simulink model "obwod_naprowadzania_JW"  (Simulink 10.2)
settings: Solver=VariableStepAuto  StartTime=0.0  StopTime=t_sim  MaxStep=0.005  EnableMultiTasking=on
values from neighbouring files (symbols this model uses):
  B_cel0 = deg2rad(-180)    [progaram_symulacyjny.m]
  E_cel0 = deg2rad(0)    [progaram_symulacyjny.m]
  v0 = 300    [progaram_symulacyjny.m]
  x0 = sqrt(23500^2-y0^2-z0^2)+v0*40    [progaram_symulacyjny.m]
  y0 = 0    [progaram_symulacyjny.m]
  z0 = 7000    [progaram_symulacyjny.m]
undefined symbols (not defined in the file or in its folder): beta_0_prim_srcp, caL, epsilon_0_prim_srcp, Fm, Fs, g, h_uwk, Im0, Im1, Is0, Is1, R, RB, RBC, RC, RE, REC, S, tm, ts, tster
libraries: simulink_extras x6, simulink x3
(part 2 of 2)

== system obwod_naprowadzania_JW/MODEL RAKIETY/Zaleznosci na skladowe sil i momentow aerodynamicznych/cx0(t) ==
  in_1 : Inport
  Constant : Constant  Value=ts
  Constant1 : Constant  Value=0.195
  Constant2 : Constant  Value=3.2
  Constant3 : Constant  Value=ts+tm
  Constant4 : Constant  Value=0.15
  Logical Operator : Logic
  Product : Product  InputSameDT=on  RndMeth=Zero  SaturateOnIntegerOverflow=on  OutDataTypeStr=Inherit: Same as first input
  Product1 : Product  InputSameDT=on  RndMeth=Zero  SaturateOnIntegerOverflow=on  OutDataTypeStr=Inherit: Same as first input
  Product2 : Product  InputSameDT=on  RndMeth=Zero  SaturateOnIntegerOverflow=on  OutDataTypeStr=Inherit: Same as first input
  Relational Operator : RelationalOperator  Operator=<=  RndMeth=Nearest  InputSameDT=on
  Relational Operator1 : RelationalOperator  Operator=>  RndMeth=Nearest  InputSameDT=on
  Relational Operator2 : RelationalOperator  Operator=<=  RndMeth=Nearest  InputSameDT=on
  Relational Operator3 : RelationalOperator  Operator=>  RndMeth=Nearest  InputSameDT=on
  Sum : Sum  Inputs=+++  InputSameDT=on  SaturateOnIntegerOverflow=on  OutDataTypeStr=Inherit: Same as first input
  out_1 : Outport
  wires:
  Sum/1 -> out_1/1
  Logical Operator/1 -> Product1/1
  Constant3/1 -> Relational Operator2/2, Relational Operator3/2
  Relational Operator2/1 -> Logical Operator/2
  Relational Operator1/1 -> Logical Operator/1
  Constant/1 -> Relational Operator1/2, Relational Operator/2
  in_1/1 -> Relational Operator1/1, Relational Operator2/1, Relational Operator3/1, Relational Operator/1
  Relational Operator/1 -> Product/2
  Constant2/1 -> Product/1
  Product/1 -> Sum/1
  Constant4/1 -> Product1/2
  Product1/1 -> Sum/2
  Relational Operator3/1 -> Product2/1
  Constant1/1 -> Product2/2
  Product2/1 -> Sum/3

== system obwod_naprowadzania_JW/MODEL RAKIETY/Zaleznosci na skladowe sil i momentow aerodynamicznych/cxi(t) ==
  in_1 : Inport
  Constant : Constant  Value=ts
  Constant2 : Constant  Value=18.9
  Constant4 : Constant  Value=5.9
  Product : Product  InputSameDT=on  RndMeth=Zero  SaturateOnIntegerOverflow=on  OutDataTypeStr=Inherit: Same as first input
  Product1 : Product  InputSameDT=on  RndMeth=Zero  SaturateOnIntegerOverflow=on  OutDataTypeStr=Inherit: Same as first input
  Relational Operator : RelationalOperator  Operator=<=  RndMeth=Nearest  InputSameDT=on
  Relational Operator1 : RelationalOperator  Operator=>  RndMeth=Nearest  InputSameDT=on
  Sum : Sum  InputSameDT=on  SaturateOnIntegerOverflow=on  OutDataTypeStr=Inherit: Same as first input
  out_1 : Outport
  wires:
  Product1/1 -> Sum/2
  Constant2/1 -> Product/1
  Relational Operator/1 -> Product/2
  in_1/1 -> Relational Operator/1, Relational Operator1/1
  Constant/1 -> Relational Operator/2, Relational Operator1/2
  Relational Operator1/1 -> Product1/1
  Sum/1 -> out_1/1
  Constant4/1 -> Product1/2
  Product/1 -> Sum/1

== system obwod_naprowadzania_JW/MODEL RAKIETY/Zaleznosci na skladowe sil i momentow aerodynamicznych/cy ==
  in_1 : Inport
  Fcn : Fcn  Expr=-u(3)*u(2)+u(4)*u(8)
  out_1 : Outport
  wires:
  Fcn/1 -> out_1/1
  in_1/1 -> Fcn/1

== system obwod_naprowadzania_JW/MODEL RAKIETY/Zaleznosci na skladowe sil i momentow aerodynamicznych/cz ==
  in_1 : Inport
  Fcn : Fcn  Expr=u(3)*u(1)+u(4)*u(7)
  out_1 : Outport
  wires:
  in_1/1 -> Fcn/1
  Fcn/1 -> out_1/1

== system obwod_naprowadzania_JW/MODEL RAKIETY/Zaleznosci na skladowe sil i momentow aerodynamicznych/cz_alfa(Ma) ==
  in_1 : Inport
  Fcn : Fcn  Expr=(0.40625-0.051875*u(1))*(180/pi)
  out_1 : Outport
  wires:
  Fcn/1 -> out_1/1
  in_1/1 -> Fcn/1

== system obwod_naprowadzania_JW/MODEL RAKIETY/Zaleznosci na skladowe sil i momentow aerodynamicznych/cz_delta(Ma) ==
  in_1 : Inport
  Fcn : Fcn  Expr=(0.02362-0.004686*u(1))*(180/pi)
  out_1 : Outport
  wires:
  in_1/1 -> Fcn/1
  Fcn/1 -> out_1/1

== system obwod_naprowadzania_JW/MODEL RAKIETY/Zaleznosci na skladowe sil i momentow aerodynamicznych/xsm(t) ==
  in_1 : Inport
  Constant : Constant  Value=ts
  Constant1 : Constant  Value=2.385
  Constant3 : Constant  Value=ts+tm
  Fcn : Fcn  Expr=3.984-((3.984-3.586)/ts)*u(1)
  Fcn1 : Fcn  Expr=2.715-((2.715-2.385)/tm)*(u(1)-ts)
  Logical Operator : Logic
  Product : Product  InputSameDT=on  RndMeth=Zero  SaturateOnIntegerOverflow=on  OutDataTypeStr=Inherit: Same as first input
  Product1 : Product  InputSameDT=on  RndMeth=Zero  SaturateOnIntegerOverflow=on  OutDataTypeStr=Inherit: Same as first input
  Product2 : Product  InputSameDT=on  RndMeth=Zero  SaturateOnIntegerOverflow=on  OutDataTypeStr=Inherit: Same as first input
  Relational Operator : RelationalOperator  Operator=<=  RndMeth=Nearest  InputSameDT=on
  Relational Operator1 : RelationalOperator  Operator=>  RndMeth=Nearest  InputSameDT=on
  Relational Operator2 : RelationalOperator  Operator=<=  RndMeth=Nearest  InputSameDT=on
  Relational Operator3 : RelationalOperator  Operator=>  RndMeth=Nearest  InputSameDT=on
  Sum : Sum  Inputs=+++  InputSameDT=on  SaturateOnIntegerOverflow=on  OutDataTypeStr=Inherit: Same as first input
  out_1 : Outport
  wires:
  Product2/1 -> Sum/3
  Constant1/1 -> Product2/2
  Relational Operator3/1 -> Product2/1
  Product1/1 -> Sum/2
  Fcn1/1 -> Product1/2
  Product/1 -> Sum/1
  Fcn/1 -> Product/1
  Relational Operator/1 -> Product/2
  in_1/1 -> Fcn/1, Relational Operator/1, Relational Operator3/1, Fcn1/1, Relational Operator2/1, Relational Operator1/1
  Constant/1 -> Relational Operator/2, Relational Operator1/2
  Relational Operator1/1 -> Logical Operator/1
  Relational Operator2/1 -> Logical Operator/2
  Constant3/1 -> Relational Operator3/2, Relational Operator2/2
  Logical Operator/1 -> Product1/1
  Sum/1 -> out_1/1

== system obwod_naprowadzania_JW/MODEL RAKIETY/Zaleznosci na skladowe sil i momentow aerodynamicznych/xsp(t) ==
  in_1 : Inport
  Constant : Constant  Value=ts
  Constant2 : Constant  Value=3.95
  Constant4 : Constant  Value=3
  Product : Product  InputSameDT=on  RndMeth=Zero  SaturateOnIntegerOverflow=on  OutDataTypeStr=Inherit: Same as first input
  Product1 : Product  InputSameDT=on  RndMeth=Zero  SaturateOnIntegerOverflow=on  OutDataTypeStr=Inherit: Same as first input
  Relational Operator : RelationalOperator  Operator=<=  RndMeth=Nearest  InputSameDT=on
  Relational Operator1 : RelationalOperator  Operator=>  RndMeth=Nearest  InputSameDT=on
  Sum : Sum  InputSameDT=on  SaturateOnIntegerOverflow=on  OutDataTypeStr=Inherit: Same as first input
  out_1 : Outport
  wires:
  Product/1 -> Sum/1
  Constant4/1 -> Product1/2
  Sum/1 -> out_1/1
  Relational Operator1/1 -> Product1/1
  Constant/1 -> Relational Operator1/2, Relational Operator/2
  in_1/1 -> Relational Operator1/1, Relational Operator/1
  Relational Operator/1 -> Product/2
  Constant2/1 -> Product/1
  Product1/1 -> Sum/2

== system obwod_naprowadzania_JW/MODEL UWK/Komendy Kierowania Waskie Pasmo/Subsystem ==
  note: f_hr1w
  hl1 : Inport
  Constant : Constant  Value=11.857142857
  Constant1 : Constant  Value=0.14
  Memory : Memory
  Product : Product  InputSameDT=on  RndMeth=Zero  SaturateOnIntegerOverflow=on  OutDataTypeStr=Inherit: Same as first input
  Product1 : Product  Inputs=*/  InputSameDT=on  RndMeth=Zero  SaturateOnIntegerOverflow=on  OutDataTypeStr=Inherit: Same as first input
  Product2 : Product  InputSameDT=on  RndMeth=Zero  SaturateOnIntegerOverflow=on  OutDataTypeStr=Inherit: Same as first input
  Product3 : Product  InputSameDT=on  RndMeth=Zero  SaturateOnIntegerOverflow=on  OutDataTypeStr=Inherit: Same as first input
  Sum : Sum  Inputs=+-  InputSameDT=on  SaturateOnIntegerOverflow=on  OutDataTypeStr=Inherit: Same as first input
  Sum1 : Sum  InputSameDT=on  SaturateOnIntegerOverflow=on  OutDataTypeStr=Inherit: Same as first input
  Sum2 : Sum  Inputs=+-  InputSameDT=on  SaturateOnIntegerOverflow=on  OutDataTypeStr=Inherit: Same as first input
  h_uwk : Constant  Value=h_uwk
  liczUR : Constant
  h1rw : Outport
  wires:
  Constant/1 -> Product/2
  Product/1 -> Sum/1, Sum2/1
  Sum/1 -> Product1/1
  Constant1/1 -> Product1/2
  Sum1/1 -> Sum/2, Memory/1, Sum2/2
  h_uwk/1 -> Product2/2
  Product1/1 -> Product2/1
  Product2/1 -> Sum1/2
  Sum2/1 -> Product3/1
  liczUR/1 -> Product3/2
  Product3/1 -> h1rw/1
  hl1/1 -> Product/1
  Memory/1 -> Sum1/1

== system obwod_naprowadzania_JW/MODEL UWK/Komendy Kierowania Waskie Pasmo/Subsystem1 ==
  hl2 : Inport
  Constant : Constant  Value=11.857142857
  Constant1 : Constant  Value=0.14
  Memory : Memory
  Product : Product  InputSameDT=on  RndMeth=Zero  SaturateOnIntegerOverflow=on  OutDataTypeStr=Inherit: Same as first input
  Product1 : Product  Inputs=*/  InputSameDT=on  RndMeth=Zero  SaturateOnIntegerOverflow=on  OutDataTypeStr=Inherit: Same as first input
  Product2 : Product  InputSameDT=on  RndMeth=Zero  SaturateOnIntegerOverflow=on  OutDataTypeStr=Inherit: Same as first input
  Product3 : Product  InputSameDT=on  RndMeth=Zero  SaturateOnIntegerOverflow=on  OutDataTypeStr=Inherit: Same as first input
  Sum : Sum  Inputs=+-  InputSameDT=on  SaturateOnIntegerOverflow=on  OutDataTypeStr=Inherit: Same as first input
  Sum1 : Sum  InputSameDT=on  SaturateOnIntegerOverflow=on  OutDataTypeStr=Inherit: Same as first input
  Sum2 : Sum  Inputs=+-  InputSameDT=on  SaturateOnIntegerOverflow=on  OutDataTypeStr=Inherit: Same as first input
  h_uwk : Constant  Value=h_uwk
  liczUR : Constant
  h2rw : Outport
  wires:
  hl2/1 -> Product/1
  Product3/1 -> h2rw/1
  liczUR/1 -> Product3/2
  Sum2/1 -> Product3/1
  Product2/1 -> Sum1/2
  Product1/1 -> Product2/1
  h_uwk/1 -> Product2/2
  Sum1/1 -> Sum2/2, Sum/2, Memory/1
  Constant1/1 -> Product1/2
  Sum/1 -> Product1/1
  Product/1 -> Sum2/1, Sum/1
  Constant/1 -> Product/2
  Memory/1 -> Sum1/1

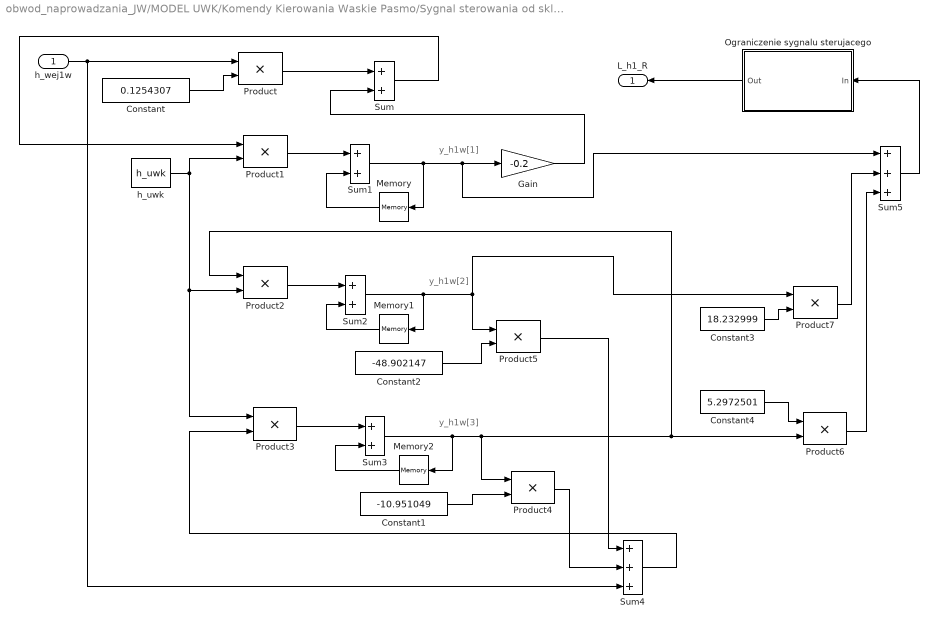
== system obwod_naprowadzania_JW/MODEL UWK/Komendy Kierowania Waskie Pasmo/Sygnal sterowania od skladowej liniowej ==
  note: y_h1w[1]
  note: y_h1w[2]
  note: y_h1w[3]
  h_wej1w : Inport
  Constant : Constant  Value=0.1254307
  Constant1 : Constant  Value=-10.951049
  Constant2 : Constant  Value=-48.902147
  Constant3 : Constant  Value=18.232999
  Constant4 : Constant  Value=5.2972501
  Gain : Gain  Gain=-0.2  SaturateOnIntegerOverflow=on  OutDataTypeStr=Inherit: Same as input  ParamDataTypeStr=Inherit: Same as input
  Memory : Memory
  Memory1 : Memory
  Memory2 : Memory
  Ograniczenie sygnalu sterujacego : Subsystem
  Product{,1..7} (8 alike) : Product  InputSameDT=on  RndMeth=Zero  SaturateOnIntegerOverflow=on  OutDataTypeStr=Inherit: Same as first input
  Sum{,1..3} (4 alike) : Sum  InputSameDT=on  SaturateOnIntegerOverflow=on  OutDataTypeStr=Inherit: Same as first input
  Sum4 : Sum  Inputs=+++  InputSameDT=on  SaturateOnIntegerOverflow=on  OutDataTypeStr=Inherit: Same as first input
  Sum5 : Sum  Inputs=+++  InputSameDT=on  SaturateOnIntegerOverflow=on  OutDataTypeStr=Inherit: Same as first input
  h_uwk : Constant  Value=h_uwk
  L_h1_R : Outport
  wires:
  h_wej1w/1 -> Product/1, Sum4/3
  Constant/1 -> Product/2
  Sum/1 -> Product1/1
  Product/1 -> Sum/1
  Sum1/1 -> Gain/1, Sum5/1, Memory/1
  h_uwk/1 -> Product1/2, Product2/2, Product3/1
  Product1/1 -> Sum1/1
  Gain/1 -> Sum/2
  Sum2/1 -> Product5/1, Product7/1, Memory1/1
  Product2/1 -> Sum2/1
  Sum3/1 -> Product4/1, Product2/1, Product6/2, Memory2/1
  Product3/1 -> Sum3/1
  Constant1/1 -> Product4/2
  Constant2/1 -> Product5/2
  Product5/1 -> Sum4/1
  Product4/1 -> Sum4/2
  Sum4/1 -> Product3/2
  Constant3/1 -> Product7/2
  Product7/1 -> Sum5/2
  Sum5/1 -> Ograniczenie sygnalu sterujacego/1(In)
  Constant4/1 -> Product6/1
  Product6/1 -> Sum5/3
  Ograniczenie sygnalu sterujacego/1(Out) -> L_h1_R/1
  Memory/1 -> Sum1/2
  Memory1/1 -> Sum2/2
  Memory2/1 -> Sum3/2

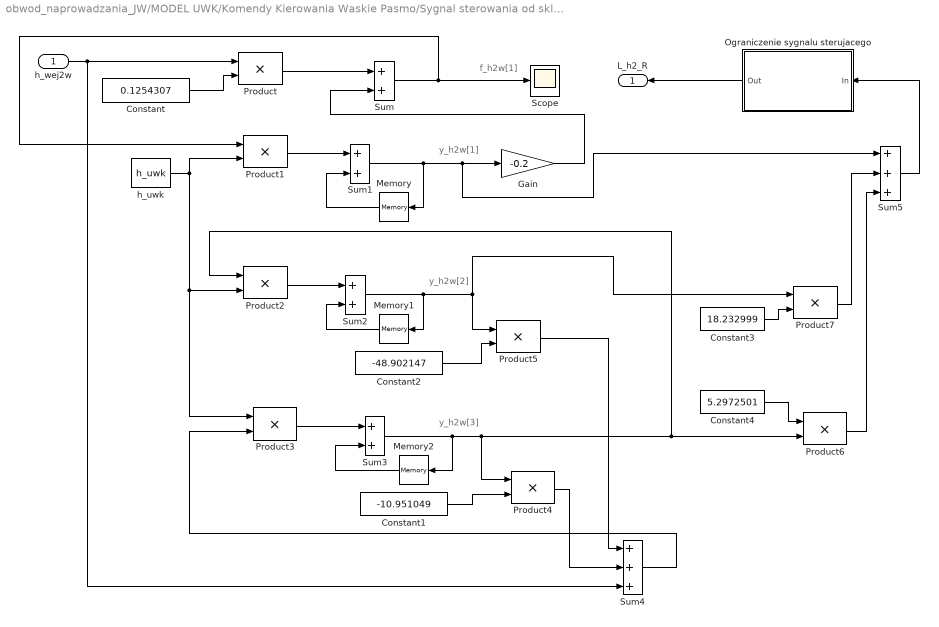
== system obwod_naprowadzania_JW/MODEL UWK/Komendy Kierowania Waskie Pasmo/Sygnal sterowania od skladowej liniowej1 ==
  note: f_h2w[1]
  note: y_h2w[3]
  note: y_h2w[2]
  note: y_h2w[1]
  h_wej2w : Inport
  Constant : Constant  Value=0.1254307
  Constant1 : Constant  Value=-10.951049
  Constant2 : Constant  Value=-48.902147
  Constant3 : Constant  Value=18.232999
  Constant4 : Constant  Value=5.2972501
  Gain : Gain  Gain=-0.2  SaturateOnIntegerOverflow=on  OutDataTypeStr=Inherit: Same as input  ParamDataTypeStr=Inherit: Same as input
  Memory : Memory
  Memory1 : Memory
  Memory2 : Memory
  Ograniczenie sygnalu sterujacego : Subsystem
  Product{,1..7} (8 alike) : Product  InputSameDT=on  RndMeth=Zero  SaturateOnIntegerOverflow=on  OutDataTypeStr=Inherit: Same as first input
  Scope : Scope
  Sum{,1..3} (4 alike) : Sum  InputSameDT=on  SaturateOnIntegerOverflow=on  OutDataTypeStr=Inherit: Same as first input
  Sum4 : Sum  Inputs=+++  InputSameDT=on  SaturateOnIntegerOverflow=on  OutDataTypeStr=Inherit: Same as first input
  Sum5 : Sum  Inputs=+++  InputSameDT=on  SaturateOnIntegerOverflow=on  OutDataTypeStr=Inherit: Same as first input
  h_uwk : Constant  Value=h_uwk
  L_h2_R : Outport
  wires:
  Memory2/1 -> Sum3/2
  Memory1/1 -> Sum2/2
  Memory/1 -> Sum1/2
  Ograniczenie sygnalu sterujacego/1(Out) -> L_h2_R/1
  Product6/1 -> Sum5/3
  Constant4/1 -> Product6/1
  Sum5/1 -> Ograniczenie sygnalu sterujacego/1(In)
  Product7/1 -> Sum5/2
  Constant3/1 -> Product7/2
  Sum4/1 -> Product3/2
  Product4/1 -> Sum4/2
  Product5/1 -> Sum4/1
  Constant2/1 -> Product5/2
  Constant1/1 -> Product4/2
  Product3/1 -> Sum3/1
  Sum3/1 -> Memory2/1, Product4/1, Product6/2, Product2/1
  Product2/1 -> Sum2/1
  Sum2/1 -> Memory1/1, Product7/1, Product5/1
  Gain/1 -> Sum/2
  Product1/1 -> Sum1/1
  h_uwk/1 -> Product3/1, Product2/2, Product1/2
  Sum1/1 -> Memory/1, Sum5/1, Gain/1
  Product/1 -> Sum/1
  Sum/1 -> Scope/1, Product1/1
  Constant/1 -> Product/2
  h_wej2w/1 -> Sum4/3, Product/1

== system obwod_naprowadzania_JW/MODEL UWK/Odchyki/gamma_R ==
  azymut : Inport
  elewacja : Inport  Port=2
  Derivative : Derivative
  Memory : Memory
  Product : Product  Inputs=4  InputSameDT=on  RndMeth=Zero  SaturateOnIntegerOverflow=on  OutDataTypeStr=Inherit: Same as first input
  Sum4 : Sum  Inputs=+-  InputSameDT=on  SaturateOnIntegerOverflow=on  OutDataTypeStr=Inherit: Same as first input
  Trigonometric Function : Trigonometry
  h_uwk : Constant  Value=h_uwk
  tster : Step  Time=tster  SampleTime=0
  gammaR : Outport
  wires:
  elewacja/1 -> Trigonometric Function/1
  Trigonometric Function/1 -> Product/2
  azymut/1 -> Derivative/1
  Derivative/1 -> Product/1
  h_uwk/1 -> Product/3
  Product/1 -> Sum4/2
  Memory/1 -> Sum4/1
  tster/1 -> Product/4
  Sum4/1 -> Memory/1, gammaR/1

== system obwod_naprowadzania_JW/MODEL CELU/Model samolotu/Ogranicznik przeciążenia  wypadkowego (max 9g)/sprzężenie zwrotne (wzrost prędkości o zadaną wartość) ==
  Fcn(n) : Inport
  u : Inport  Port=2
  -Fcn(n) : Inport  Port=3
  y : Inport  Port=4
  Add : Sum  Inputs=+-
  Add1 : Sum
  Gain1 : Gain  Gain=-1
  Integrator : Integrator
  Integrator1 : Integrator
  Switch : Switch  Criteria=u2 > Threshold  Threshold=0.000001
  Switch1 : Switch  Criteria=u2 > Threshold  Threshold=0.000001
  Zero : Constant  Value=0  OutDataTypeStr=Inherit: Inherit via back propagation
  Zero1 : Constant  Value=0  OutDataTypeStr=Inherit: Inherit via back propagation
  sprz : Outport
  wires:
  Integrator/1 -> Add/2
  Add/1 -> Gain1/1, Switch/2
  Zero/1 -> Switch/3
  Integrator1/1 -> Add/1
  Gain1/1 -> Switch1/2
  Zero1/1 -> Switch1/3
  Switch/1 -> Add1/1
  Switch1/1 -> Add1/2
  Fcn(n)/1 -> Switch/1
  u/1 -> Integrator1/1
  y/1 -> Integrator/1
  Add1/1 -> sprz/1
  -Fcn(n)/1 -> Switch1/1

== system obwod_naprowadzania_JW/MODEL CELU/Model samolotu/Ogranicznik przeciążenia azymut (max 4g)/sprzężenie zwrotne (skręt o zadany kąt) ==
  u : Inport
  Fcn(v) : Inport  Port=2
  y : Inport  Port=3
  Add : Sum  Inputs=+-
  Add1 : Sum
  Gain1 : Gain  Gain=-1
  Gain2 : Gain  Gain=-1
  Integrator : Integrator
  Integrator1 : Integrator
  Switch : Switch  Criteria=u2 > Threshold  Threshold=0.000001
  Switch1 : Switch  Criteria=u2 > Threshold  Threshold=0.000001
  Zero : Constant  Value=0  OutDataTypeStr=Inherit: Inherit via back propagation
  Zero1 : Constant  Value=0  OutDataTypeStr=Inherit: Inherit via back propagation
  sprz : Outport
  wires:
  Integrator/1 -> Add/2
  Add/1 -> Gain1/1, Switch/2
  Zero/1 -> Switch/3
  Integrator1/1 -> Add/1
  Gain1/1 -> Switch1/2
  Zero1/1 -> Switch1/3
  Switch/1 -> Add1/1
  Gain2/1 -> Switch1/1
  Switch1/1 -> Add1/2
  Fcn(v)/1 -> Switch/1, Gain2/1
  u/1 -> Integrator1/1
  y/1 -> Integrator/1
  Add1/1 -> sprz/1

== system obwod_naprowadzania_JW/MODEL CELU/Model samolotu/Ogranicznik przeciążenia elewacja (max 8g)/sprzężenie zwrotne (skręt o zadany kąt) ==
  u : Inport
  Fcn(v) : Inport  Port=2
  y : Inport  Port=3
  Add : Sum  Inputs=+-
  Add1 : Sum
  Gain1 : Gain  Gain=-1
  Gain2 : Gain  Gain=-1
  Integrator : Integrator
  Integrator1 : Integrator
  Switch : Switch  Criteria=u2 > Threshold  Threshold=0.000001
  Switch1 : Switch  Criteria=u2 > Threshold  Threshold=0.000001
  Zero : Constant  Value=0  OutDataTypeStr=Inherit: Inherit via back propagation
  Zero1 : Constant  Value=0  OutDataTypeStr=Inherit: Inherit via back propagation
  Out1 : Outport
  wires:
  Integrator/1 -> Add/2
  Add/1 -> Gain1/1, Switch/2
  Zero/1 -> Switch/3
  Integrator1/1 -> Add/1
  Gain1/1 -> Switch1/2
  Zero1/1 -> Switch1/3
  Switch/1 -> Add1/1
  Gain2/1 -> Switch1/1
  Switch1/1 -> Add1/2
  Fcn(v)/1 -> Switch/1, Gain2/1
  u/1 -> Integrator1/1
  y/1 -> Integrator/1
  Add1/1 -> Out1/1

== system obwod_naprowadzania_JW/MODEL RAKIETY/Zaleznosci na skladowe sil i momentow aerodynamicznych/PN-78/N-03100  /cisnienie ==
  H : Inport
  11000 > H >= 0 : Subsystem
  20000 > H >= 11000 : Subsystem
  32000 > H >= 20000 : Subsystem
  47000 > H >= 32000 : Subsystem
  51000 > H >= 47000 : Subsystem
  71000 > H >= 51000 : Subsystem
  80000 > H >= 71000 : Subsystem
  Sum : Sum  Inputs=+++++++  InputSameDT=on  SaturateOnIntegerOverflow=on  OutDataTypeStr=Inherit: Same as first input
  "cisnienie - p [Pa] " : Scope
  p : Outport
  wires:
  80000 > H >= 71000/1(Out1) -> Sum/7
  71000 > H >= 51000/1(Out1) -> Sum/6
  51000 > H >= 47000/1(Out1) -> Sum/5
  47000 > H >= 32000/1(Out1) -> Sum/4
  32000 > H >= 20000/1(Out1) -> Sum/3
  20000 > H >= 11000/1(Out1) -> Sum/2
  Sum/1 -> "cisnienie - p [Pa] "/1, p/1
  11000 > H >= 0/1(Out1) -> Sum/1
  H/1 -> 80000 > H >= 71000/1(In1), 71000 > H >= 51000/1(In1), 51000 > H >= 47000/1(In1), 47000 > H >= 32000/1(In1), 32000 > H >= 20000/1(In1), 20000 > H >= 11000/1(In1), 11000 > H >= 0/1(In1)

== system obwod_naprowadzania_JW/MODEL RAKIETY/Zaleznosci na skladowe sil i momentow aerodynamicznych/PN-78/N-03100  /gestosc ==
  note: wlasciwa stala gazowa - R
  p : Inport
  T : Inport  Port=2
  Math Function : Math  Operator=reciprocal  SignedPower=on  SaturateOnIntegerOverflow=on
  Product1 : Product  InputSameDT=on  RndMeth=Zero  SaturateOnIntegerOverflow=on  OutDataTypeStr=Inherit: Same as first input
  Product2 : Product  InputSameDT=on  RndMeth=Zero  SaturateOnIntegerOverflow=on  OutDataTypeStr=Inherit: Same as first input
  R [J/K*kg] [m2/K*s2] : Constant  Value=287.05287
  "gestosc [kg/m3] " : Scope
  gestosc : Outport
  wires:
  Product2/1 -> "gestosc [kg/m3] "/1, gestosc/1
  p/1 -> Product2/1
  Math Function/1 -> Product2/2
  Product1/1 -> Math Function/1
  T/1 -> Product1/1
  R [J/K*kg] [m2/K*s2]/1 -> Product1/2

== system obwod_naprowadzania_JW/MODEL RAKIETY/Zaleznosci na skladowe sil i momentow aerodynamicznych/PN-78/N-03100  /predkosc dzwieku ==
  note: wlasciwa stala gazowa - R
  note: wykladnik adiabaty - stosunek ciepla wlasciwego
      | powietrza przy stalym cisnieniu do jego ciepla
      | wlasciwego przy stalej objetosci
  note: temperatura termodynamiczna - T [K]
  T : Inport
  Math Function : Math  Operator=sqrt  SignedPower=on  SaturateOnIntegerOverflow=on
  Math Function1 : Math  Operator=sqrt  SignedPower=on  SaturateOnIntegerOverflow=on
  Product : Product  InputSameDT=on  RndMeth=Zero  SaturateOnIntegerOverflow=on  OutDataTypeStr=Inherit: Same as first input
  Product1 : Product  Inputs=3  InputSameDT=on  RndMeth=Zero  SaturateOnIntegerOverflow=on  OutDataTypeStr=Inherit: Same as first input
  R [J/K*kg] [m2/K*s2] : Constant  Value=287.05287
  k=Cp/Cv : Constant  Value=1.4
  "predkosc dzwieku - a [m/s] " : Scope
  predkosc dzwieku a [m/s] : Scope
  stala : Constant  Value=20.046796
  predkosc dzwieku : Outport
  wires:
  Product1/1 -> Math Function1/1
  R [J/K*kg] [m2/K*s2]/1 -> Product1/2
  k=Cp/Cv/1 -> Product1/1
  Math Function1/1 -> predkosc dzwieku a [m/s]/1, predkosc dzwieku/1
  Product/1 -> "predkosc dzwieku - a [m/s] "/1
  stala/1 -> Product/2
  Math Function/1 -> Product/1
  T/1 -> Product1/3, Math Function/1

== system obwod_naprowadzania_JW/MODEL RAKIETY/Zaleznosci na skladowe sil i momentow aerodynamicznych/PN-78/N-03100  /temperatura termodynamiczna ==
  note: wysokosc geopotencjalna - H [m]
  note: temperatura termodynamiczna
      | punktu topnienia lodu
      | pod cisnieniem 101325,0 Pa
  H : Inport
  Look-Up Table : Lookup  InputValues=[-2000 0 11000 20000 32000 47000 51000 71000 80000]  Table=[301.15 288.15 216.65 216.65 228.65 270.65 270.65 214.65 196.65]  SaturateOnIntegerOverflow=on
  Saturation : Saturate  UpperLimit=80000  LowerLimit=-2000
  Sum : Sum  Inputs=-+  InputSameDT=on  SaturateOnIntegerOverflow=on  OutDataTypeStr=Inherit: Same as first input
  T[oC] : Scope
  To [K] : Constant  Value=273.15
  "temperatura termodynamiczna - T [K] " : Scope
  T : Outport
  wires:
  Sum/1 -> T[oC]/1
  To [K]/1 -> Sum/1
  Look-Up Table/1 -> "temperatura termodynamiczna - T [K] "/1, T/1, Sum/2
  Saturation/1 -> Look-Up Table/1
  H/1 -> Saturation/1

== system obwod_naprowadzania_JW/MODEL RAKIETY/Zaleznosci na skladowe sil i momentow aerodynamicznych/PN-78/N-03100  /wysokosc geopotencjalna i przyspieszenie ==
  note: wysokosc geometryczna - h [m]
  h : Inport
  Math Function : Math  Operator=reciprocal  SignedPower=on  SaturateOnIntegerOverflow=on
  Math Function1 : Math  Operator=square  SignedPower=on  SaturateOnIntegerOverflow=on
  Product{,1..3} (4 alike) : Product  InputSameDT=on  RndMeth=Zero  SaturateOnIntegerOverflow=on  OutDataTypeStr=Inherit: Same as first input
  Sum : Sum  InputSameDT=on  SaturateOnIntegerOverflow=on  OutDataTypeStr=Inherit: Same as first input
  nominalny promien ziemi - r [m] : Constant  Value=6356766
  przyspieszenie - g [m/s2] : Scope
  wysokosc geopotencjalna - H [m] : Scope
  wzorcowe przyspieszenie przy swobodnym spadku - gn [m/s2] : Constant  Value=9.80665
  H : Outport
  wires:
  Product3/1 -> H/1, wysokosc geopotencjalna - H [m]/1
  Product2/1 -> Product3/2
  Product1/1 -> przyspieszenie - g [m/s2]/1
  Math Function1/1 -> Product1/1
  wzorcowe przyspieszenie przy swobodnym spadku - gn [m/s2]/1 -> Product1/2
  Product/1 -> Math Function1/1
  Math Function/1 -> Product3/1, Product/2
  Sum/1 -> Math Function/1
  h/1 -> Product2/2, Sum/2
  nominalny promien ziemi - r [m]/1 -> Product2/1, Product/1, Sum/1

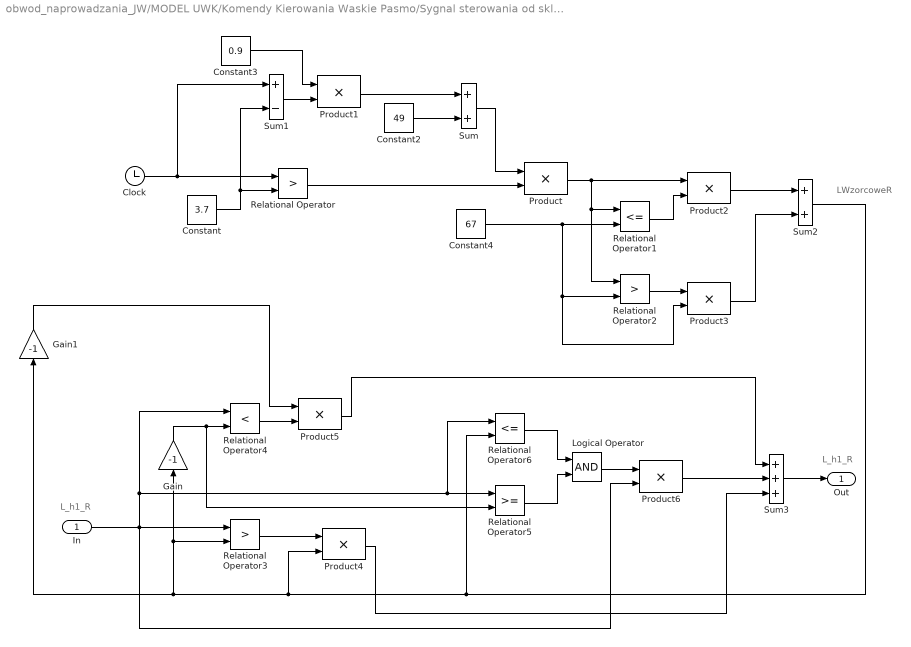
== system obwod_naprowadzania_JW/MODEL UWK/Komendy Kierowania Waskie Pasmo/Sygnal sterowania od skladowej liniowej/Ograniczenie sygnalu sterujacego ==
  note: LWzorcoweR
  note: L_h1_R
  note: L_h1_R
  In : Inport
  Clock : Clock
  Constant : Constant  Value=3.7
  Constant2 : Constant  Value=49
  Constant3 : Constant  Value=0.9
  Constant4 : Constant  Value=67
  Gain : Gain  Gain=-1  SaturateOnIntegerOverflow=on  OutDataTypeStr=Inherit: Same as input  ParamDataTypeStr=Inherit: Same as input
  Gain1 : Gain  Gain=-1  SaturateOnIntegerOverflow=on  OutDataTypeStr=Inherit: Same as input  ParamDataTypeStr=Inherit: Same as input
  Logical Operator : Logic
  Product{,1..6} (7 alike) : Product  InputSameDT=on  RndMeth=Zero  SaturateOnIntegerOverflow=on  OutDataTypeStr=Inherit: Same as first input
  Relational Operator : RelationalOperator  Operator=>  RndMeth=Nearest  InputSameDT=on
  Relational Operator1 : RelationalOperator  Operator=<=  RndMeth=Nearest  InputSameDT=on
  Relational Operator2 : RelationalOperator  Operator=>  RndMeth=Nearest  InputSameDT=on
  Relational Operator3 : RelationalOperator  Operator=>  RndMeth=Nearest  InputSameDT=on
  Relational Operator4 : RelationalOperator  Operator=<  RndMeth=Nearest  InputSameDT=on
  Relational Operator5 : RelationalOperator  RndMeth=Nearest  InputSameDT=on
  Relational Operator6 : RelationalOperator  Operator=<=  RndMeth=Nearest  InputSameDT=on
  Sum : Sum  InputSameDT=on  SaturateOnIntegerOverflow=on  OutDataTypeStr=Inherit: Same as first input
  Sum1 : Sum  Inputs=+-  InputSameDT=on  SaturateOnIntegerOverflow=on  OutDataTypeStr=Inherit: Same as first input
  Sum2 : Sum  InputSameDT=on  SaturateOnIntegerOverflow=on  OutDataTypeStr=Inherit: Same as first input
  Sum3 : Sum  Inputs=+++  InputSameDT=on  SaturateOnIntegerOverflow=on  OutDataTypeStr=Inherit: Same as first input
  Out : Outport
  wires:
  Clock/1 -> Relational Operator/1, Sum1/1
  Constant/1 -> Relational Operator/2, Sum1/2
  Constant2/1 -> Sum/2
  Sum1/1 -> Product1/2
  Constant3/1 -> Product1/1
  Product1/1 -> Sum/1
  Sum/1 -> Product/1
  Relational Operator/1 -> Product/2
  Sum2/1 -> Product4/2, Relational Operator3/2, Gain/1, Gain1/1, Relational Operator6/2
  Constant4/1 -> Relational Operator1/2, Relational Operator2/2, Product3/2
  Product/1 -> Product2/1, Relational Operator1/1, Relational Operator2/1
  Relational Operator1/1 -> Product2/2
  Product2/1 -> Sum2/1
  Relational Operator2/1 -> Product3/1
  Product3/1 -> Sum2/2
  In/1 -> Relational Operator3/1, Relational Operator4/1, Relational Operator5/1, Relational Operator6/1, Product6/2
  Relational Operator3/1 -> Product4/1
  Product4/1 -> Sum3/3
  Gain/1 -> Relational Operator4/2, Relational Operator5/2
  Relational Operator4/1 -> Product5/2
  Gain1/1 -> Product5/1
  Product5/1 -> Sum3/1
  Relational Operator5/1 -> Logical Operator/2
  Relational Operator6/1 -> Logical Operator/1
  Logical Operator/1 -> Product6/1
  Product6/1 -> Sum3/2
  Sum3/1 -> Out/1

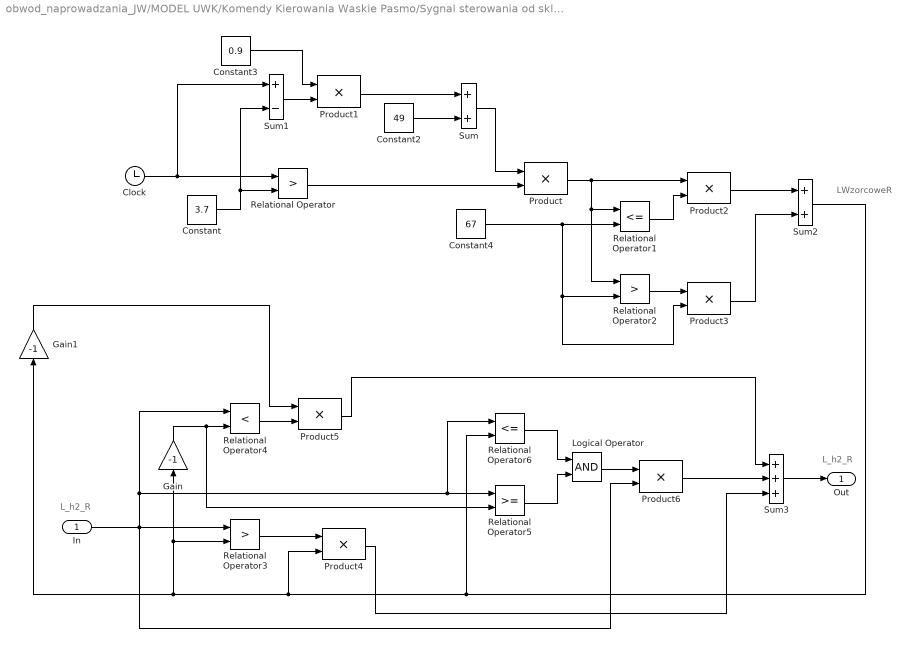
== system obwod_naprowadzania_JW/MODEL UWK/Komendy Kierowania Waskie Pasmo/Sygnal sterowania od skladowej liniowej1/Ograniczenie sygnalu sterujacego ==
  note: L_h2_R
  note: L_h2_R
  note: LWzorcoweR
  In : Inport
  Clock : Clock
  Constant : Constant  Value=3.7
  Constant2 : Constant  Value=49
  Constant3 : Constant  Value=0.9
  Constant4 : Constant  Value=67
  Gain : Gain  Gain=-1  SaturateOnIntegerOverflow=on  OutDataTypeStr=Inherit: Same as input  ParamDataTypeStr=Inherit: Same as input
  Gain1 : Gain  Gain=-1  SaturateOnIntegerOverflow=on  OutDataTypeStr=Inherit: Same as input  ParamDataTypeStr=Inherit: Same as input
  Logical Operator : Logic
  Product{,1..6} (7 alike) : Product  InputSameDT=on  RndMeth=Zero  SaturateOnIntegerOverflow=on  OutDataTypeStr=Inherit: Same as first input
  Relational Operator : RelationalOperator  Operator=>  RndMeth=Nearest  InputSameDT=on
  Relational Operator1 : RelationalOperator  Operator=<=  RndMeth=Nearest  InputSameDT=on
  Relational Operator2 : RelationalOperator  Operator=>  RndMeth=Nearest  InputSameDT=on
  Relational Operator3 : RelationalOperator  Operator=>  RndMeth=Nearest  InputSameDT=on
  Relational Operator4 : RelationalOperator  Operator=<  RndMeth=Nearest  InputSameDT=on
  Relational Operator5 : RelationalOperator  RndMeth=Nearest  InputSameDT=on
  Relational Operator6 : RelationalOperator  Operator=<=  RndMeth=Nearest  InputSameDT=on
  Sum : Sum  InputSameDT=on  SaturateOnIntegerOverflow=on  OutDataTypeStr=Inherit: Same as first input
  Sum1 : Sum  Inputs=+-  InputSameDT=on  SaturateOnIntegerOverflow=on  OutDataTypeStr=Inherit: Same as first input
  Sum2 : Sum  InputSameDT=on  SaturateOnIntegerOverflow=on  OutDataTypeStr=Inherit: Same as first input
  Sum3 : Sum  Inputs=+++  InputSameDT=on  SaturateOnIntegerOverflow=on  OutDataTypeStr=Inherit: Same as first input
  Out : Outport
  wires:
  Sum3/1 -> Out/1
  Product6/1 -> Sum3/2
  Logical Operator/1 -> Product6/1
  Relational Operator6/1 -> Logical Operator/1
  Relational Operator5/1 -> Logical Operator/2
  Product5/1 -> Sum3/1
  Gain1/1 -> Product5/1
  Relational Operator4/1 -> Product5/2
  Gain/1 -> Relational Operator5/2, Relational Operator4/2
  Product4/1 -> Sum3/3
  Relational Operator3/1 -> Product4/1
  In/1 -> Product6/2, Relational Operator6/1, Relational Operator5/1, Relational Operator4/1, Relational Operator3/1
  Product3/1 -> Sum2/2
  Relational Operator2/1 -> Product3/1
  Product2/1 -> Sum2/1
  Relational Operator1/1 -> Product2/2
  Product/1 -> Relational Operator2/1, Relational Operator1/1, Product2/1
  Constant4/1 -> Product3/2, Relational Operator2/2, Relational Operator1/2
  Sum2/1 -> Relational Operator6/2, Gain1/1, Gain/1, Relational Operator3/2, Product4/2
  Relational Operator/1 -> Product/2
  Sum/1 -> Product/1
  Product1/1 -> Sum/1
  Constant3/1 -> Product1/1
  Sum1/1 -> Product1/2
  Constant2/1 -> Sum/2
  Constant/1 -> Sum1/2, Relational Operator/2
  Clock/1 -> Sum1/1, Relational Operator/1

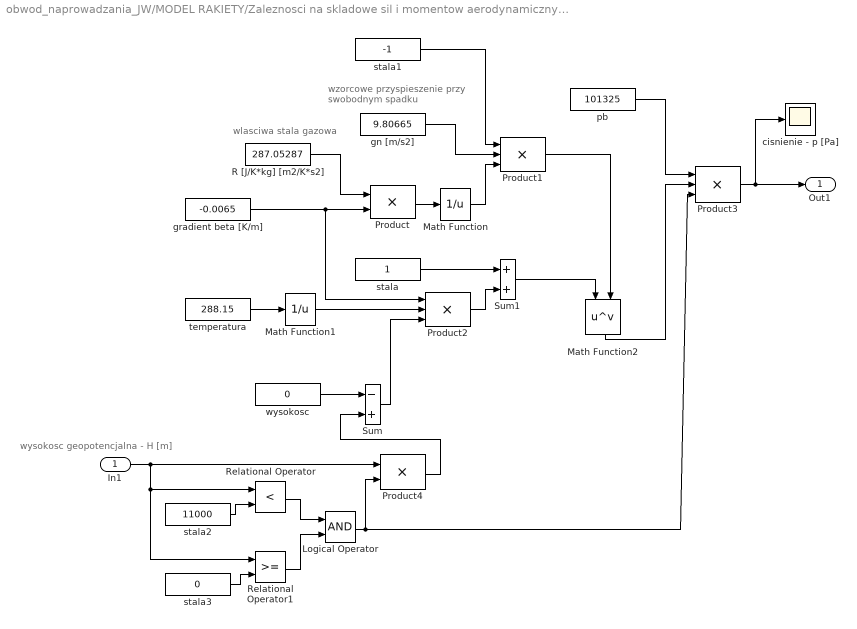
== system obwod_naprowadzania_JW/MODEL RAKIETY/Zaleznosci na skladowe sil i momentow aerodynamicznych/PN-78/N-03100  /cisnienie/11000 > H >= 0 ==
  note: wlasciwa stala gazowa
  note: wzorcowe przyspieszenie przy
      | swobodnym spadku
  note: wysokosc geopotencjalna - H [m]
  In1 : Inport
  Logical Operator : Logic
  Math Function : Math  Operator=reciprocal  SignedPower=on  SaturateOnIntegerOverflow=on
  Math Function1 : Math  Operator=reciprocal  SignedPower=on  SaturateOnIntegerOverflow=on
  Math Function2 : Math  Operator=pow  SignedPower=on  SaturateOnIntegerOverflow=on
  Product : Product  InputSameDT=on  RndMeth=Zero  SaturateOnIntegerOverflow=on  OutDataTypeStr=Inherit: Same as first input
  Product1 : Product  Inputs=3  InputSameDT=on  RndMeth=Zero  SaturateOnIntegerOverflow=on  OutDataTypeStr=Inherit: Same as first input
  Product2 : Product  Inputs=3  InputSameDT=on  RndMeth=Zero  SaturateOnIntegerOverflow=on  OutDataTypeStr=Inherit: Same as first input
  Product3 : Product  Inputs=3  InputSameDT=on  RndMeth=Zero  SaturateOnIntegerOverflow=on  OutDataTypeStr=Inherit: Same as first input
  Product4 : Product  InputSameDT=on  RndMeth=Zero  SaturateOnIntegerOverflow=on  OutDataTypeStr=Inherit: Same as first input
  R [J/K*kg] [m2/K*s2] : Constant  Value=287.05287
  Relational Operator : RelationalOperator  Operator=<  RndMeth=Nearest  InputSameDT=on
  Relational Operator1 : RelationalOperator  RndMeth=Nearest  InputSameDT=on
  Sum : Sum  Inputs=-+  InputSameDT=on  SaturateOnIntegerOverflow=on  OutDataTypeStr=Inherit: Same as first input
  Sum1 : Sum  InputSameDT=on  SaturateOnIntegerOverflow=on  OutDataTypeStr=Inherit: Same as first input
  "cisnienie - p [Pa] " : Scope
  gn [m/s2] : Constant  Value=9.80665
  gradient beta [K/m] : Constant  Value=-0.0065
  pb : Constant  Value=101325
  stala : Constant
  stala1 : Constant  Value=-1
  stala2 : Constant  Value=11000
  stala3 : Constant  Value=0
  temperatura : Constant  Value=288.15
  wysokosc : Constant  Value=0
  Out1 : Outport
  wires:
  In1/1 -> Product4/1, Relational Operator1/1, Relational Operator/1
  Product4/1 -> Sum/2
  Logical Operator/1 -> Product3/3, Product4/2
  Relational Operator/1 -> Logical Operator/1
  Relational Operator1/1 -> Logical Operator/2
  stala3/1 -> Relational Operator1/2
  stala2/1 -> Relational Operator/2
  Product1/1 -> Math Function2/2
  Sum1/1 -> Math Function2/1
  Product3/1 -> Out1/1, "cisnienie - p [Pa] "/1
  Math Function2/1 -> Product3/2
  pb/1 -> Product3/1
  Product2/1 -> Sum1/2
  stala/1 -> Sum1/1
  Sum/1 -> Product2/3
  wysokosc/1 -> Sum/1
  Math Function1/1 -> Product2/2
  temperatura/1 -> Math Function1/1
  stala1/1 -> Product1/1
  gn [m/s2]/1 -> Product1/2
  Math Function/1 -> Product1/3
  Product/1 -> Math Function/1
  R [J/K*kg] [m2/K*s2]/1 -> Product/1
  gradient beta [K/m]/1 -> Product2/1, Product/2

== system obwod_naprowadzania_JW/MODEL RAKIETY/Zaleznosci na skladowe sil i momentow aerodynamicznych/PN-78/N-03100  /cisnienie/20000 > H >= 11000 ==
  note: wysokosc geopotencjalna - H [m]
  note: wzorcowe przyspieszenie przy
      | swobodnym spadku
  note: wlasciwa stala gazowa
  In1 : Inport
  Logical Operator : Logic
  Math Function : Math  Operator=reciprocal  SignedPower=on  SaturateOnIntegerOverflow=on
  Math Function1 : Math  SignedPower=on  SaturateOnIntegerOverflow=on
  Product : Product  InputSameDT=on  RndMeth=Zero  SaturateOnIntegerOverflow=on  OutDataTypeStr=Inherit: Same as first input
  Product1 : Product  Inputs=4  InputSameDT=on  RndMeth=Zero  SaturateOnIntegerOverflow=on  OutDataTypeStr=Inherit: Same as first input
  Product3 : Product  Inputs=3  InputSameDT=on  RndMeth=Zero  SaturateOnIntegerOverflow=on  OutDataTypeStr=Inherit: Same as first input
  Product4 : Product  InputSameDT=on  RndMeth=Zero  SaturateOnIntegerOverflow=on  OutDataTypeStr=Inherit: Same as first input
  R [J/K*kg] [m2/K*s2] : Constant  Value=287.05287
  Relational Operator : RelationalOperator  Operator=<  RndMeth=Nearest  InputSameDT=on
  Relational Operator1 : RelationalOperator  RndMeth=Nearest  InputSameDT=on
  Sum : Sum  Inputs=-+  InputSameDT=on  SaturateOnIntegerOverflow=on  OutDataTypeStr=Inherit: Same as first input
  T : Constant  Value=216.65
  "cisnienie - p [Pa] " : Scope
  gn [m/s2] : Constant  Value=9.80665
  pb : Constant  Value=22700
  stala1 : Constant  Value=-1
  stala2 : Constant  Value=20000
  stala3 : Constant  Value=11000
  wysokosc : Constant  Value=11000
  Out1 : Outport
  wires:
  Math Function1/1 -> Product3/2
  Product1/1 -> Math Function1/1
  T/1 -> Product/2
  R [J/K*kg] [m2/K*s2]/1 -> Product/1
  Product/1 -> Math Function/1
  Math Function/1 -> Product1/3
  gn [m/s2]/1 -> Product1/2
  stala1/1 -> Product1/1
  wysokosc/1 -> Sum/1
  Sum/1 -> Product1/4
  pb/1 -> Product3/1
  Product3/1 -> Out1/1, "cisnienie - p [Pa] "/1
  stala2/1 -> Relational Operator/2
  stala3/1 -> Relational Operator1/2
  Relational Operator1/1 -> Logical Operator/2
  Relational Operator/1 -> Logical Operator/1
  Logical Operator/1 -> Product4/2, Product3/3
  Product4/1 -> Sum/2
  In1/1 -> Relational Operator/1, Relational Operator1/1, Product4/1

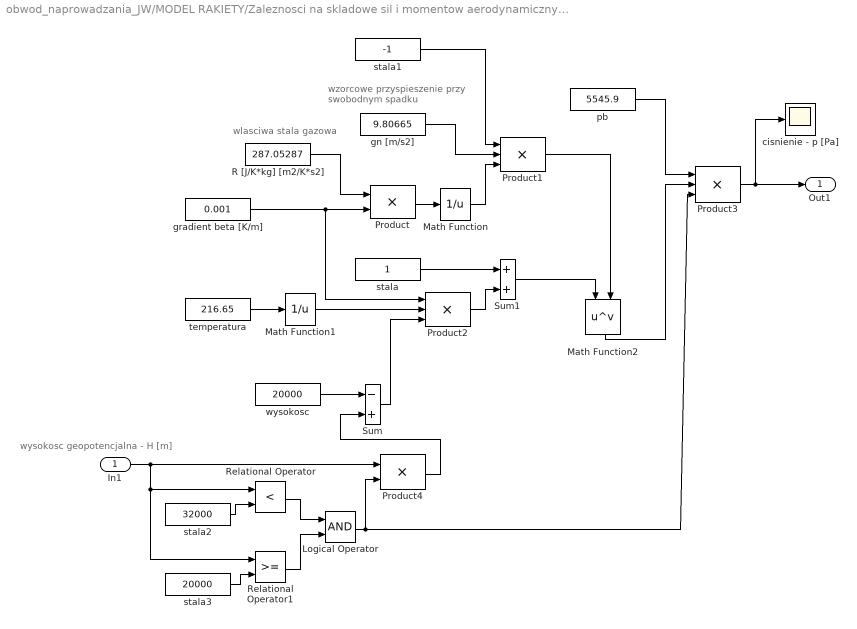
== system obwod_naprowadzania_JW/MODEL RAKIETY/Zaleznosci na skladowe sil i momentow aerodynamicznych/PN-78/N-03100  /cisnienie/32000 > H >= 20000 ==
  note: wlasciwa stala gazowa
  note: wzorcowe przyspieszenie przy
      | swobodnym spadku
  note: wysokosc geopotencjalna - H [m]
  In1 : Inport
  Logical Operator : Logic
  Math Function : Math  Operator=reciprocal  SignedPower=on  SaturateOnIntegerOverflow=on
  Math Function1 : Math  Operator=reciprocal  SignedPower=on  SaturateOnIntegerOverflow=on
  Math Function2 : Math  Operator=pow  SignedPower=on  SaturateOnIntegerOverflow=on
  Product : Product  InputSameDT=on  RndMeth=Zero  SaturateOnIntegerOverflow=on  OutDataTypeStr=Inherit: Same as first input
  Product1 : Product  Inputs=3  InputSameDT=on  RndMeth=Zero  SaturateOnIntegerOverflow=on  OutDataTypeStr=Inherit: Same as first input
  Product2 : Product  Inputs=3  InputSameDT=on  RndMeth=Zero  SaturateOnIntegerOverflow=on  OutDataTypeStr=Inherit: Same as first input
  Product3 : Product  Inputs=3  InputSameDT=on  RndMeth=Zero  SaturateOnIntegerOverflow=on  OutDataTypeStr=Inherit: Same as first input
  Product4 : Product  InputSameDT=on  RndMeth=Zero  SaturateOnIntegerOverflow=on  OutDataTypeStr=Inherit: Same as first input
  R [J/K*kg] [m2/K*s2] : Constant  Value=287.05287
  Relational Operator : RelationalOperator  Operator=<  RndMeth=Nearest  InputSameDT=on
  Relational Operator1 : RelationalOperator  RndMeth=Nearest  InputSameDT=on
  Sum : Sum  Inputs=-+  InputSameDT=on  SaturateOnIntegerOverflow=on  OutDataTypeStr=Inherit: Same as first input
  Sum1 : Sum  InputSameDT=on  SaturateOnIntegerOverflow=on  OutDataTypeStr=Inherit: Same as first input
  "cisnienie - p [Pa] " : Scope
  gn [m/s2] : Constant  Value=9.80665
  gradient beta [K/m] : Constant  Value=0.001
  pb : Constant  Value=5545.9
  stala : Constant
  stala1 : Constant  Value=-1
  stala2 : Constant  Value=32000
  stala3 : Constant  Value=20000
  temperatura : Constant  Value=216.65
  wysokosc : Constant  Value=20000
  Out1 : Outport
  wires:
  In1/1 -> Product4/1, Relational Operator1/1, Relational Operator/1
  Product4/1 -> Sum/2
  Logical Operator/1 -> Product3/3, Product4/2
  Relational Operator/1 -> Logical Operator/1
  Relational Operator1/1 -> Logical Operator/2
  stala3/1 -> Relational Operator1/2
  stala2/1 -> Relational Operator/2
  Product1/1 -> Math Function2/2
  Sum1/1 -> Math Function2/1
  Product3/1 -> Out1/1, "cisnienie - p [Pa] "/1
  Math Function2/1 -> Product3/2
  pb/1 -> Product3/1
  Product2/1 -> Sum1/2
  stala/1 -> Sum1/1
  Sum/1 -> Product2/3
  wysokosc/1 -> Sum/1
  Math Function1/1 -> Product2/2
  temperatura/1 -> Math Function1/1
  stala1/1 -> Product1/1
  gn [m/s2]/1 -> Product1/2
  Math Function/1 -> Product1/3
  Product/1 -> Math Function/1
  R [J/K*kg] [m2/K*s2]/1 -> Product/1
  gradient beta [K/m]/1 -> Product2/1, Product/2

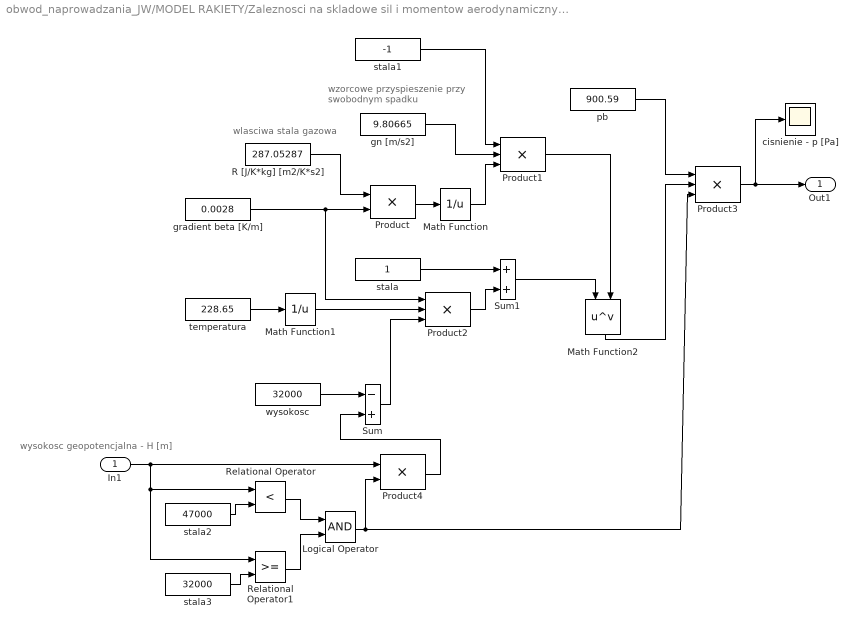
== system obwod_naprowadzania_JW/MODEL RAKIETY/Zaleznosci na skladowe sil i momentow aerodynamicznych/PN-78/N-03100  /cisnienie/47000 > H >= 32000 ==
  note: wysokosc geopotencjalna - H [m]
  note: wzorcowe przyspieszenie przy
      | swobodnym spadku
  note: wlasciwa stala gazowa
  In1 : Inport
  Logical Operator : Logic
  Math Function : Math  Operator=reciprocal  SignedPower=on  SaturateOnIntegerOverflow=on
  Math Function1 : Math  Operator=reciprocal  SignedPower=on  SaturateOnIntegerOverflow=on
  Math Function2 : Math  Operator=pow  SignedPower=on  SaturateOnIntegerOverflow=on
  Product : Product  InputSameDT=on  RndMeth=Zero  SaturateOnIntegerOverflow=on  OutDataTypeStr=Inherit: Same as first input
  Product1 : Product  Inputs=3  InputSameDT=on  RndMeth=Zero  SaturateOnIntegerOverflow=on  OutDataTypeStr=Inherit: Same as first input
  Product2 : Product  Inputs=3  InputSameDT=on  RndMeth=Zero  SaturateOnIntegerOverflow=on  OutDataTypeStr=Inherit: Same as first input
  Product3 : Product  Inputs=3  InputSameDT=on  RndMeth=Zero  SaturateOnIntegerOverflow=on  OutDataTypeStr=Inherit: Same as first input
  Product4 : Product  InputSameDT=on  RndMeth=Zero  SaturateOnIntegerOverflow=on  OutDataTypeStr=Inherit: Same as first input
  R [J/K*kg] [m2/K*s2] : Constant  Value=287.05287
  Relational Operator : RelationalOperator  Operator=<  RndMeth=Nearest  InputSameDT=on
  Relational Operator1 : RelationalOperator  RndMeth=Nearest  InputSameDT=on
  Sum : Sum  Inputs=-+  InputSameDT=on  SaturateOnIntegerOverflow=on  OutDataTypeStr=Inherit: Same as first input
  Sum1 : Sum  InputSameDT=on  SaturateOnIntegerOverflow=on  OutDataTypeStr=Inherit: Same as first input
  "cisnienie - p [Pa] " : Scope
  gn [m/s2] : Constant  Value=9.80665
  gradient beta [K/m] : Constant  Value=0.0028
  pb : Constant  Value=900.59
  stala : Constant
  stala1 : Constant  Value=-1
  stala2 : Constant  Value=47000
  stala3 : Constant  Value=32000
  temperatura : Constant  Value=228.65
  wysokosc : Constant  Value=32000
  Out1 : Outport
  wires:
  gradient beta [K/m]/1 -> Product/2, Product2/1
  R [J/K*kg] [m2/K*s2]/1 -> Product/1
  Product/1 -> Math Function/1
  Math Function/1 -> Product1/3
  gn [m/s2]/1 -> Product1/2
  stala1/1 -> Product1/1
  temperatura/1 -> Math Function1/1
  Math Function1/1 -> Product2/2
  wysokosc/1 -> Sum/1
  Sum/1 -> Product2/3
  stala/1 -> Sum1/1
  Product2/1 -> Sum1/2
  pb/1 -> Product3/1
  Math Function2/1 -> Product3/2
  Product3/1 -> "cisnienie - p [Pa] "/1, Out1/1
  Sum1/1 -> Math Function2/1
  Product1/1 -> Math Function2/2
  stala2/1 -> Relational Operator/2
  stala3/1 -> Relational Operator1/2
  Relational Operator1/1 -> Logical Operator/2
  Relational Operator/1 -> Logical Operator/1
  Logical Operator/1 -> Product4/2, Product3/3
  Product4/1 -> Sum/2
  In1/1 -> Relational Operator/1, Relational Operator1/1, Product4/1

== system obwod_naprowadzania_JW/MODEL RAKIETY/Zaleznosci na skladowe sil i momentow aerodynamicznych/PN-78/N-03100  /cisnienie/51000 > H >= 47000 ==
  note: wlasciwa stala gazowa
  note: wzorcowe przyspieszenie przy
      | swobodnym spadku
  note: wysokosc geopotencjalna - H [m]
  In1 : Inport
  Logical Operator : Logic
  Math Function : Math  Operator=reciprocal  SignedPower=on  SaturateOnIntegerOverflow=on
  Math Function1 : Math  SignedPower=on  SaturateOnIntegerOverflow=on
  Product : Product  InputSameDT=on  RndMeth=Zero  SaturateOnIntegerOverflow=on  OutDataTypeStr=Inherit: Same as first input
  Product1 : Product  Inputs=4  InputSameDT=on  RndMeth=Zero  SaturateOnIntegerOverflow=on  OutDataTypeStr=Inherit: Same as first input
  Product3 : Product  Inputs=3  InputSameDT=on  RndMeth=Zero  SaturateOnIntegerOverflow=on  OutDataTypeStr=Inherit: Same as first input
  Product4 : Product  InputSameDT=on  RndMeth=Zero  SaturateOnIntegerOverflow=on  OutDataTypeStr=Inherit: Same as first input
  R [J/K*kg] [m2/K*s2] : Constant  Value=287.05287
  Relational Operator : RelationalOperator  Operator=<  RndMeth=Nearest  InputSameDT=on
  Relational Operator1 : RelationalOperator  RndMeth=Nearest  InputSameDT=on
  Sum : Sum  Inputs=-+  InputSameDT=on  SaturateOnIntegerOverflow=on  OutDataTypeStr=Inherit: Same as first input
  T : Constant  Value=270.65
  "cisnienie - p [Pa] " : Scope
  gn [m/s2] : Constant  Value=9.80665
  pb : Constant  Value=120.2
  stala1 : Constant  Value=-1
  stala2 : Constant  Value=51000
  stala3 : Constant  Value=47000
  wysokosc : Constant  Value=47000
  Out1 : Outport
  wires:
  In1/1 -> Product4/1, Relational Operator1/1, Relational Operator/1
  Product4/1 -> Sum/2
  Logical Operator/1 -> Product3/3, Product4/2
  Relational Operator/1 -> Logical Operator/1
  Relational Operator1/1 -> Logical Operator/2
  stala3/1 -> Relational Operator1/2
  stala2/1 -> Relational Operator/2
  Product3/1 -> "cisnienie - p [Pa] "/1, Out1/1
  pb/1 -> Product3/1
  Sum/1 -> Product1/4
  wysokosc/1 -> Sum/1
  stala1/1 -> Product1/1
  gn [m/s2]/1 -> Product1/2
  Math Function/1 -> Product1/3
  Product/1 -> Math Function/1
  R [J/K*kg] [m2/K*s2]/1 -> Product/1
  T/1 -> Product/2
  Product1/1 -> Math Function1/1
  Math Function1/1 -> Product3/2

== system obwod_naprowadzania_JW/MODEL RAKIETY/Zaleznosci na skladowe sil i momentow aerodynamicznych/PN-78/N-03100  /cisnienie/71000 > H >= 51000 ==
  note: wlasciwa stala gazowa
  note: wzorcowe przyspieszenie przy
      | swobodnym spadku
  note: wysokosc geopotencjalna - H [m]
  In1 : Inport
  Logical Operator : Logic
  Math Function : Math  Operator=reciprocal  SignedPower=on  SaturateOnIntegerOverflow=on
  Math Function1 : Math  Operator=reciprocal  SignedPower=on  SaturateOnIntegerOverflow=on
  Math Function2 : Math  Operator=pow  SignedPower=on  SaturateOnIntegerOverflow=on
  Product : Product  InputSameDT=on  RndMeth=Zero  SaturateOnIntegerOverflow=on  OutDataTypeStr=Inherit: Same as first input
  Product1 : Product  Inputs=3  InputSameDT=on  RndMeth=Zero  SaturateOnIntegerOverflow=on  OutDataTypeStr=Inherit: Same as first input
  Product2 : Product  Inputs=3  InputSameDT=on  RndMeth=Zero  SaturateOnIntegerOverflow=on  OutDataTypeStr=Inherit: Same as first input
  Product3 : Product  Inputs=3  InputSameDT=on  RndMeth=Zero  SaturateOnIntegerOverflow=on  OutDataTypeStr=Inherit: Same as first input
  Product4 : Product  InputSameDT=on  RndMeth=Zero  SaturateOnIntegerOverflow=on  OutDataTypeStr=Inherit: Same as first input
  R [J/K*kg] [m2/K*s2] : Constant  Value=287.05287
  Relational Operator : RelationalOperator  Operator=<  RndMeth=Nearest  InputSameDT=on
  Relational Operator1 : RelationalOperator  RndMeth=Nearest  InputSameDT=on
  Sum : Sum  Inputs=-+  InputSameDT=on  SaturateOnIntegerOverflow=on  OutDataTypeStr=Inherit: Same as first input
  Sum1 : Sum  InputSameDT=on  SaturateOnIntegerOverflow=on  OutDataTypeStr=Inherit: Same as first input
  "cisnienie - p [Pa] " : Scope
  gn [m/s2] : Constant  Value=9.80665
  gradient beta [K/m] : Constant  Value=-0.0028
  pb : Constant  Value=76.362
  stala : Constant
  stala1 : Constant  Value=-1
  stala2 : Constant  Value=71000
  stala3 : Constant  Value=51000
  temperatura : Constant  Value=270.65
  wysokosc : Constant  Value=51000
  Out1 : Outport
  wires:
  In1/1 -> Product4/1, Relational Operator1/1, Relational Operator/1
  Product4/1 -> Sum/2
  Logical Operator/1 -> Product3/3, Product4/2
  Relational Operator/1 -> Logical Operator/1
  Relational Operator1/1 -> Logical Operator/2
  stala3/1 -> Relational Operator1/2
  stala2/1 -> Relational Operator/2
  Product1/1 -> Math Function2/2
  Sum1/1 -> Math Function2/1
  Product3/1 -> Out1/1, "cisnienie - p [Pa] "/1
  Math Function2/1 -> Product3/2
  pb/1 -> Product3/1
  Product2/1 -> Sum1/2
  stala/1 -> Sum1/1
  Sum/1 -> Product2/3
  wysokosc/1 -> Sum/1
  Math Function1/1 -> Product2/2
  temperatura/1 -> Math Function1/1
  stala1/1 -> Product1/1
  gn [m/s2]/1 -> Product1/2
  Math Function/1 -> Product1/3
  Product/1 -> Math Function/1
  R [J/K*kg] [m2/K*s2]/1 -> Product/1
  gradient beta [K/m]/1 -> Product2/1, Product/2

== system obwod_naprowadzania_JW/MODEL RAKIETY/Zaleznosci na skladowe sil i momentow aerodynamicznych/PN-78/N-03100  /cisnienie/80000 > H >= 71000 ==
  note: wysokosc geopotencjalna - H [m]
  note: wzorcowe przyspieszenie przy
      | swobodnym spadku
  note: wlasciwa stala gazowa
  In1 : Inport
  Logical Operator : Logic
  Math Function : Math  Operator=reciprocal  SignedPower=on  SaturateOnIntegerOverflow=on
  Math Function1 : Math  Operator=reciprocal  SignedPower=on  SaturateOnIntegerOverflow=on
  Math Function2 : Math  Operator=pow  SignedPower=on  SaturateOnIntegerOverflow=on
  Product : Product  InputSameDT=on  RndMeth=Zero  SaturateOnIntegerOverflow=on  OutDataTypeStr=Inherit: Same as first input
  Product1 : Product  Inputs=3  InputSameDT=on  RndMeth=Zero  SaturateOnIntegerOverflow=on  OutDataTypeStr=Inherit: Same as first input
  Product2 : Product  Inputs=3  InputSameDT=on  RndMeth=Zero  SaturateOnIntegerOverflow=on  OutDataTypeStr=Inherit: Same as first input
  Product3 : Product  Inputs=3  InputSameDT=on  RndMeth=Zero  SaturateOnIntegerOverflow=on  OutDataTypeStr=Inherit: Same as first input
  Product4 : Product  InputSameDT=on  RndMeth=Zero  SaturateOnIntegerOverflow=on  OutDataTypeStr=Inherit: Same as first input
  R [J/K*kg] [m2/K*s2] : Constant  Value=287.05287
  Relational Operator : RelationalOperator  Operator=<  RndMeth=Nearest  InputSameDT=on
  Relational Operator1 : RelationalOperator  RndMeth=Nearest  InputSameDT=on
  Sum : Sum  Inputs=-+  InputSameDT=on  SaturateOnIntegerOverflow=on  OutDataTypeStr=Inherit: Same as first input
  Sum1 : Sum  InputSameDT=on  SaturateOnIntegerOverflow=on  OutDataTypeStr=Inherit: Same as first input
  "cisnienie - p [Pa] " : Scope
  gn [m/s2] : Constant  Value=9.80665
  gradient beta [K/m] : Constant  Value=-0.002
  pb : Constant  Value=5.1102
  stala : Constant
  stala1 : Constant  Value=-1
  stala2 : Constant  Value=80000
  stala3 : Constant  Value=71000
  temperatura : Constant  Value=214.65
  wysokosc : Constant  Value=71000
  Out1 : Outport
  wires:
  gradient beta [K/m]/1 -> Product/2, Product2/1
  R [J/K*kg] [m2/K*s2]/1 -> Product/1
  Product/1 -> Math Function/1
  Math Function/1 -> Product1/3
  gn [m/s2]/1 -> Product1/2
  stala1/1 -> Product1/1
  temperatura/1 -> Math Function1/1
  Math Function1/1 -> Product2/2
  wysokosc/1 -> Sum/1
  Sum/1 -> Product2/3
  stala/1 -> Sum1/1
  Product2/1 -> Sum1/2
  pb/1 -> Product3/1
  Math Function2/1 -> Product3/2
  Product3/1 -> "cisnienie - p [Pa] "/1, Out1/1
  Sum1/1 -> Math Function2/1
  Product1/1 -> Math Function2/2
  stala2/1 -> Relational Operator/2
  stala3/1 -> Relational Operator1/2
  Relational Operator1/1 -> Logical Operator/2
  Relational Operator/1 -> Logical Operator/1
  Logical Operator/1 -> Product4/2, Product3/3
  Product4/1 -> Sum/2
  In1/1 -> Relational Operator/1, Relational Operator1/1, Product4/1

== matlab function WARUNKI SYMULACJI/MATLAB Function ==
  data: dR input double; y output double; R input double
function y = fcn(dR,R)
if dR > 0 || R < 15
    y=1;
else
    y=0;
end
end
